simulink model "lnl_working3"  (R2020a)
settings: Solver=VariableStepAuto  StartTime=0  StopTime=40  MaxStep=0.01  RelTol=1e-3
libraries: simulink x1
settings Model: Creator=Peter  LastModifiedBy=Peter

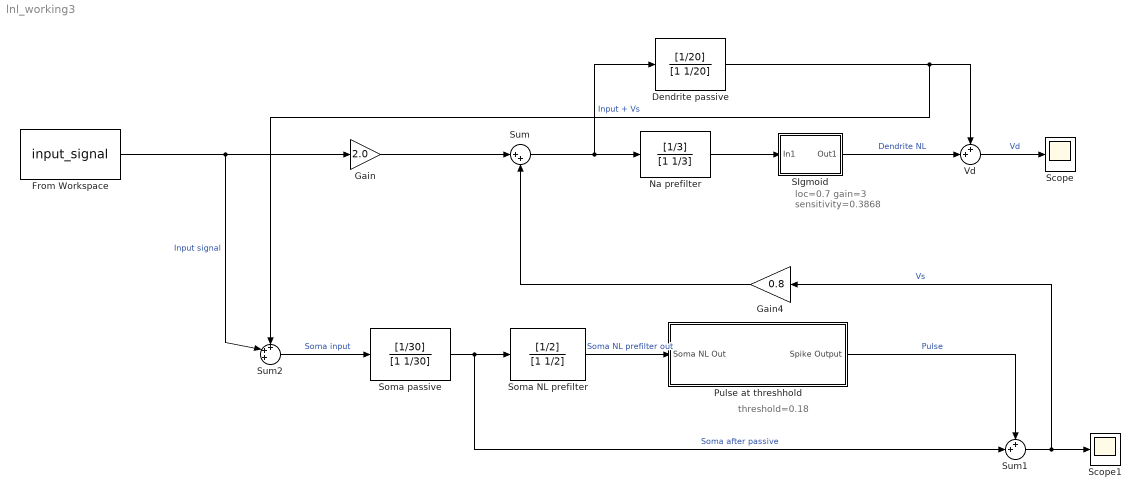
== system lnl_working3 ==
  note: threshold=0.18
  note: loc=0.7
      | gain=3
      | sensitivity=0.3868
  Dendrite passive : TransferFcn  Numerator=[1/20]  Denominator=[1 1/20]
  From Workspace : FromWorkspace  VariableName=input_signal
  Gain : Gain  Gain=2.0
  Gain4 : Gain  Gain=0.8
  Na prefilter : TransferFcn  Numerator=[1/3]  Denominator=[1 1/3]
  Pulse at threshhold : Subsystem
  SIgmoid : Subsystem  mask{Loc=1.7, Gain=3, Sensitivity=0.3868}
      mask TypeOptions Loc: loc/Value
      mask TypeOptions Gain: Gain1/Gain
      mask TypeOptions Sensitivity: sensitivity/Value
  Scope : Scope
  Scope1 : Scope
  Soma NL prefilter : TransferFcn  Numerator=[1/2]  Denominator=[1 1/2]
  Soma passive : TransferFcn  Numerator=[1/30]  Denominator=[1 1/30]
  Sum : Sum  Inputs=|++
  Sum1 : Sum  Inputs=++|
  Sum2 : Sum  Inputs=+++|
  Vd : Sum  Inputs=++|
  wires:
  Na prefilter/1 -> SIgmoid/1(In1)
  SIgmoid/1(Out1) -> Vd/2  "Dendrite NL"
  Dendrite passive/1 -> Sum2/1, Vd/1
  Vd/1 -> Scope/1  "Vd"
  Sum/1 -> Dendrite passive/1, Na prefilter/1  "Input + Vs"
  Soma passive/1 -> Soma NL prefilter/1, Sum1/2  "Soma after passive"
  Sum1/1 -> Gain4/1, Scope1/1  "Vs"
  Gain4/1 -> Sum/2
  Pulse at threshhold/1(Spike Output) -> Sum1/1  "Pulse"
  Soma NL prefilter/1 -> Pulse at threshhold/1(Soma NL Out)  "Soma NL prefilter out"
  Sum2/1 -> Soma passive/1  "Soma input"
  Gain/1 -> Sum/1
  From Workspace/1 -> Sum2/2, Gain/1  "Input signal"

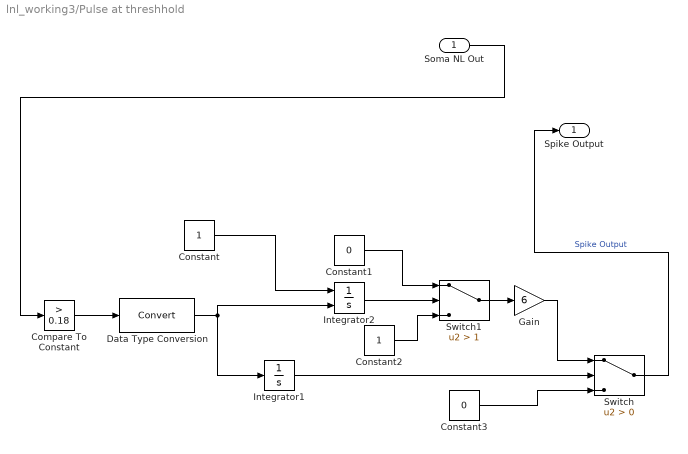
== system lnl_working3/Pulse at threshhold ==
  Soma NL Out : Inport
  Compare To Constant : simulink/Logic and Bit Operations/Compare To Constant  relop=>  const=0.18  OutDataTypeStr=boolean
  Constant : Constant
  Constant1 : Constant  Value=0
  Constant2 : Constant
  Constant3 : Constant  Value=0
  Data Type Conversion : DataTypeConversion  RndMeth=Round
  Gain : Gain  Gain=6
  Integrator1 : Integrator
  Integrator2 : Integrator  ExternalReset=rising
  Switch : Switch  Criteria=u2 > Threshold
  Switch1 : Switch  Criteria=u2 > Threshold  Threshold=1
  Spike Output : Outport
  wires:
  Integrator1/1 -> Switch/2
  Compare To Constant/1 -> Data Type Conversion/1
  Data Type Conversion/1 -> Integrator1/1, Integrator2/2
  Soma NL Out/1 -> Compare To Constant/1
  Switch/1 -> Spike Output/1  "Spike Output"
  Constant/1 -> Integrator2/1
  Integrator2/1 -> Switch1/2
  Constant2/1 -> Switch1/3
  Constant1/1 -> Switch1/1
  Constant3/1 -> Switch/3
  Switch1/1 -> Gain/1
  Gain/1 -> Switch/1

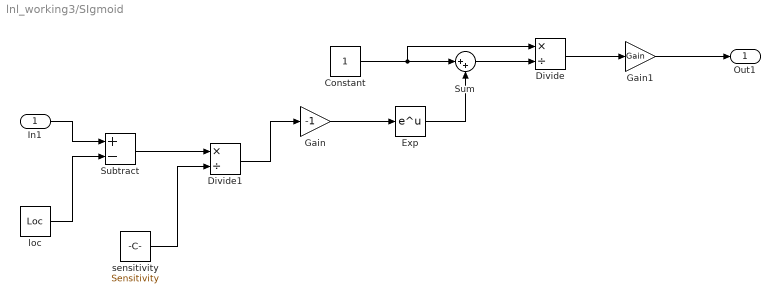
== system lnl_working3/SIgmoid ==
  In1 : Inport
  Constant : Constant
  Divide : Product  Inputs=*/
  Divide1 : Product  Inputs=*/
  Exp : Math  SaturateOnIntegerOverflow=on
  Gain : Gain  Gain=-1
  Gain1 : Gain  Gain=Gain
  Subtract : Sum  Inputs=+-
  Sum : Sum  Inputs=|++
  loc : Constant  Value=Loc
  sensitivity : Constant  Value=Sensitivity
  Out1 : Outport
  wires:
  Gain/1 -> Exp/1
  Constant/1 -> Divide/1, Sum/1
  Exp/1 -> Sum/2
  Sum/1 -> Divide/2
  In1/1 -> Subtract/1
  loc/1 -> Subtract/2
  Subtract/1 -> Divide1/1
  sensitivity/1 -> Divide1/2
  Divide1/1 -> Gain/1
  Divide/1 -> Gain1/1
  Gain1/1 -> Out1/1
